simulink model "theta_control_robutst"  (R2019b)
settings: Solver=VariableStepAuto  StartTime=0.0  StopTime=10  RelTol=1e-3
values from neighbouring files (symbols this model uses):
  aa = 6.945 + 6.945*(rand()-0.5)*2*0.4    [robustness_check.m]
  bb = 14.29 + 14.29*(rand()-0.5)*2*0.4    [robustness_check.m]
settings Model: Creator=JianFongLee  LastModifiedBy=JianFongLee

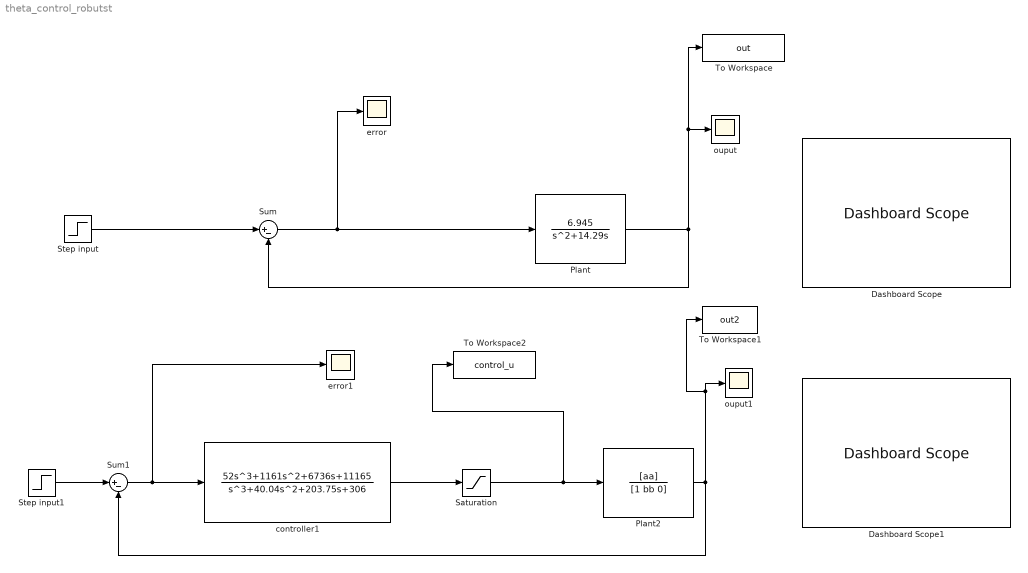
== system theta_control_robutst ==
  " Plant" : TransferFcn  Numerator=[6.945]  Denominator=[1 14.29 0]
  " Plant2" : TransferFcn  Numerator=[aa]  Denominator=[1 bb 0]
  Dashboard Scope : DashboardScope
  Dashboard Scope1 : DashboardScope
  Saturation : Saturate  UpperLimit=12  LowerLimit=-12
  Step input : Step  Time=0  SampleTime=0
  Step input1 : Step  Time=0  SampleTime=0
  Sum : Sum  Inputs=|+-
  Sum1 : Sum  Inputs=|+-
  To Workspace : ToWorkspace  VariableName=out  SaveFormat=Timeseries  SampleTime=-1
  To Workspace1 : ToWorkspace  VariableName=out2  SaveFormat=Timeseries  SampleTime=-1
  To Workspace2 : ToWorkspace  VariableName=control_u  SaveFormat=Timeseries  SampleTime=-1
  controller1 : TransferFcn  Numerator=[52 1161 6736 11165]  Denominator=[1 40.04 203.75 306]
  error : Scope
  error1 : Scope
  ouput : Scope
  ouput1 : Scope
  wires:
  Step input/1 -> Sum/1
  Sum/1 -> error/1, " Plant"/1
  " Plant"/1 -> Sum/2, To Workspace/1, ouput/1
  " Plant2"/1 -> Sum1/2, To Workspace1/1, ouput1/1
  Sum1/1 -> controller1/1, error1/1
  Step input1/1 -> Sum1/1
  controller1/1 -> Saturation/1
  Saturation/1 -> To Workspace2/1, " Plant2"/1
